simulink model "model_sym"  (R2016a)
settings: Solver=ode45  StartTime=0.0  StopTime=T  MaxStep=0.5  MinStep=0.4  RelTol=1e-3
undefined symbols (not defined in the file): A, b, c, d, M
settings Model: Creator=student  LastModifiedBy=Radosław
settings DataIOCC: LimitDataPoints=on  SaveFormat=Array  SignalLoggingSaveFormat=ModelDataLogs
settings OptimizationCC: ExpressionDepthLimit=2147483647
settings DebuggingCC: UnderspecifiedInitializationDetection=Classic  MergeDetectMultiDrivingBlocksExec=none  SolverPrmCheckMsg=warning  FcnCallInpInsideContextMsg=EnableAllAsWarning  UnknownTsInhSupMsg=none  StateNameClashWarn=warning
settings HardwareCC: ProdBitPerPointer=32  ProdLargestAtomicFloat=None  ProdIntDivRoundTo=Undefined  ProdEndianess=Unspecified  ProdWordSize=32  ProdHWDeviceType=32-bit Generic
settings ModelReferenceCC: PropagateSignalLabelsOutOfModel=off
settings ConfigComp: CovModelRefEnable=Off

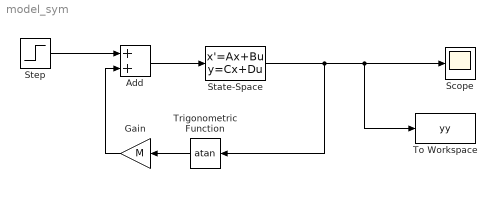
== system model_sym ==
  Add : Sum
  Gain : Gain  Gain=M
  Scope : Scope
  State-Space : StateSpace  A=A  B=b  C=c  D=d  X0=0
  Step : Step  Time=0  SampleTime=0
  To Workspace : ToWorkspace  VariableName=yy  SampleTime=-1
  Trigonometric Function : Trigonometry  Operator=atan
  wires:
  Trigonometric Function/1 -> Gain/1
  Step/1 -> Add/1
  Add/1 -> State-Space/1
  State-Space/1 -> Trigonometric Function/1, To Workspace/1, Scope/1
  Gain/1 -> Add/2
